simulink model "Model_7"  (R2020b)
settings: Solver=VariableStepAuto  StartTime=0.0  StopTime=10.0  RelTol=1e-3
settings Model: Creator=samar  LastModifiedBy=samar

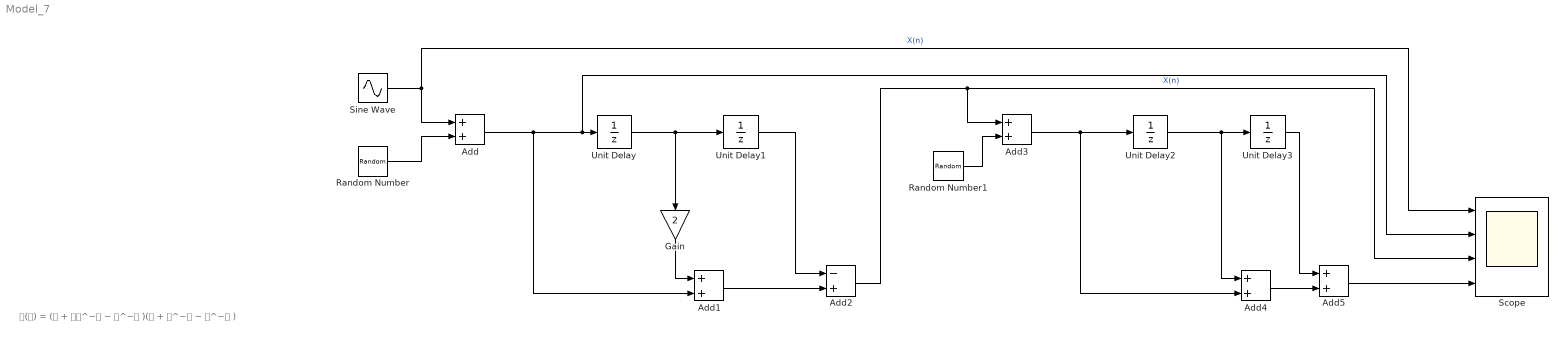
== system Model_7 ==
  note: 𝐇(𝐳) = (𝟏 + 𝟐𝐳^−𝟏 − 𝐳^−𝟐 )(𝟏 + 𝐳^−𝟏 − 𝐳^−𝟐 )
  Add{,1,3..5} (5 alike) : Sum
  Add2 : Sum  Inputs=-+
  Gain : Gain  Gain=2
  Random Number : RandomNumber  Mean=1  Variance=0.01  SampleTime=0.1
  Random Number1 : RandomNumber  Mean=1  Variance=0.01  SampleTime=0.1
  Scope : Scope  NumInputPorts=4
  Sine Wave : Sin  SampleTime=0
  Unit Delay{,1..3} (4 alike) : UnitDelay  SampleTime=-1  HasFrameUpgradeWarning=on
  wires:
  Sine Wave/1 -> Add/1, Scope/1  "X(n)"
  Add/1 -> Scope/2, Unit Delay/1, Add1/2
  Unit Delay/1 -> Gain/1, Unit Delay1/1
  Unit Delay1/1 -> Add2/1
  Gain/1 -> Add1/1
  Add1/1 -> Add2/2
  Random Number/1 -> Add/2
  Random Number1/1 -> Add3/2
  Add3/1 -> Add4/2, Unit Delay2/1
  Add2/1 -> Add3/1, Scope/3  "X(n)"
  Unit Delay3/1 -> Add5/1
  Add4/1 -> Add5/2
  Unit Delay2/1 -> Add4/1, Unit Delay3/1
  Add5/1 -> Scope/4
